simulink model "AC_Capacity_Estimation_Model_AT"  (R2024a)
settings: Solver=FixedStepAuto  StartTime=503  StopTime=2309  FixedStep=0.1  RelTol=1e-3
values from neighbouring files (symbols this model uses):
  airDensity = 1.165    [AC_Capacity_Estimation_Model_Parameters.m]
  airDragCoeff = 0.558    [AC_Capacity_Estimation_Model_Parameters.m]
  frontalArea = 0.958    [AC_Capacity_Estimation_Model_Parameters.m]
  g = 9.8    [AC_Capacity_Estimation_Model_Parameters.m]
  rollingResistCoeff = 0.030    (= 0.03)    [AC_Capacity_Estimation_Model_Parameters.m]
  vehicleMass = 284    [AC_Capacity_Estimation_Model_Parameters.m]
settings Model: Creator=salaz  LastModifiedBy=aimee
settings RTWCC: GPUComputeCapability=3.5

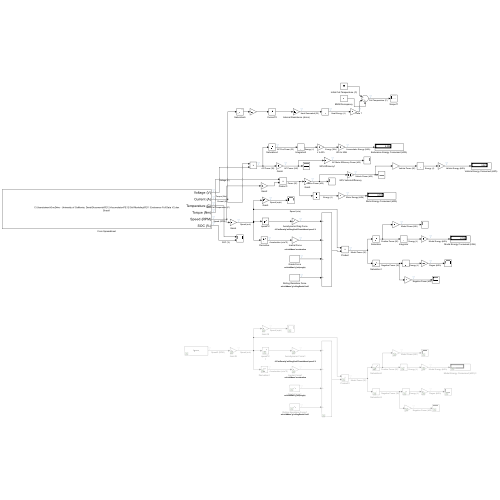
[thumbnail: Simulink's stored preview of the top-level diagram]
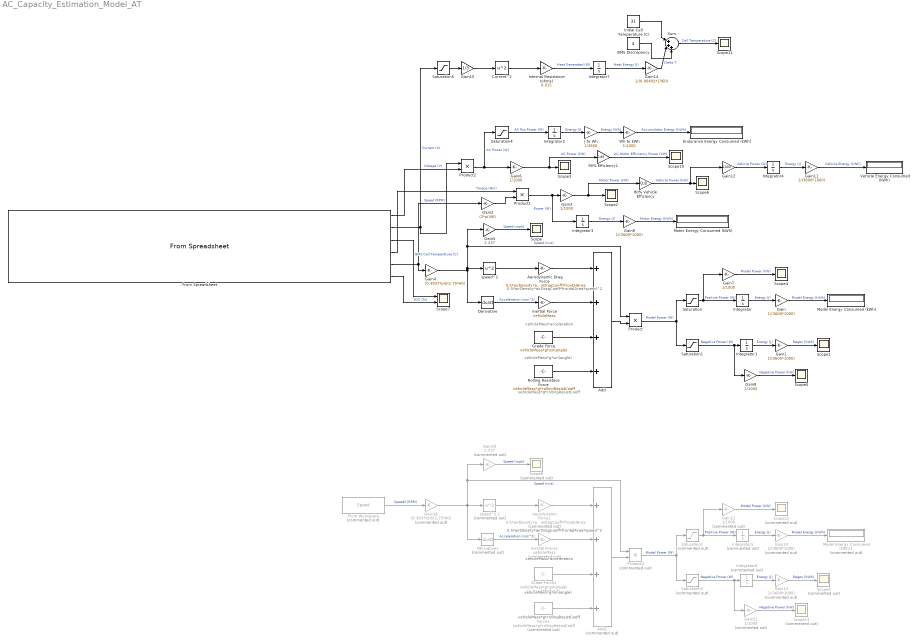
== system AC_Capacity_Estimation_Model_AT ==
  note: 0.5*airDensity*airDragCoeff*frontalArea*speed^2
  note: vehicleMass*acceleration
  note: vehicleMass*g*sin(angle)
  note: vehicleMass*g*rollingResistCoeff
  note: 0.5*airDensity*airDragCoeff*frontalArea*speed^2
  note: vehicleMass*acceleration
  note: vehicleMass*g*sin(angle)
  note: vehicleMass*g*rollingResistCoeff
  80% Vehicle Efficiency : Gain  Gain=0.8
  90% Efficiency1 : Gain  Gain=0.85
  Add : Sum  Inputs=++++
  Add1 : Sum  Commented=on  Inputs=++++
  Aerodynamic Drag Force : Gain  Gain=0.5*airDensity*airDragCoeff*frontalArea
  Aerodynamic Force1 : Gain  Commented=on  Gain=0.5*airDensity*airDragCoeff*frontalArea
  BMS Discrepancy : Constant  Value=4
  "Current^2 " : Math  Operator=square
  Derivative : Derivative
  Derivative1 : Derivative  Commented=on
  "Endurance Energy Consumed (kWh) " : Display
  From Workspace : FromWorkspace  Commented=on  VariableName=Speed
  From Spreadsheet : FromSpreadsheet  FileName=C:\Users\aimee\OneDrive - University of California, Davis\Documents\FE12-Accumulator\FE12\Cell Modeling\FE11 Endurance Full Data V2.xlsx
  Gain{,1,9,11} (4 alike) : Gain  Gain=1/(3600*1000)
  Gain10 : Gain  Commented=on  Gain=1/(3600*1000)
  Gain12 : Gain  Gain=1000
  Gain13 : Gain  Commented=on  Gain=1/(3600*1000)
  Gain14 : Gain  Gain=1/(0.06492*1360)
  Gain15 : Gain  Gain=1/3
  Gain18 : Gain  Commented=on  Gain=(0.3937*pi)/(2.75*60)
  Gain19 : Gain  Commented=on  Gain=2.237
  Gain2 : Gain  Gain=(2*pi)/60
  Gain21 : Gain  Commented=on  Gain=1/1000
  Gain22 : Gain  Commented=on  Gain=1/1000
  Gain{3,6..8} (4 alike) : Gain  Gain=1/1000
  Gain4 : Gain  Gain=(0.3937*pi)/(2.75*60)
  Gain5 : Gain  Gain=2.237
  Grade Force : Constant  Value=vehicleMass*g*sin(angle)
  Grade Force1 : Constant  Commented=on  Value=vehicleMass*g*sin(angle)
  Inertial Force : Gain  Gain=vehicleMass
  Inertial Force1 : Gain  Commented=on  Gain=vehicleMass
  Initial Cell Temperature (C) : Constant  Value=31
  Integrator{,1..4,7} (6 alike) : Integrator
  Integrator5 : Integrator  Commented=on
  Integrator6 : Integrator  Commented=on
  Internal Resistance (ohms) : Gain  Gain=0.015
  J to Wh : Gain  Gain=1/3600
  Model Energy Consumed (kWh) : Display
  Model Energy Consumed (kWh)1 : Display  Commented=on
  Motor Energy Consumed (kWh) : Display
  Product : Product
  Product1 : Product
  Product2 : Product
  Product3 : Product  Commented=on
  Rolling Resistace Force : Constant  Value=vehicleMass*g*rollingResistCoeff
  Rolling Resistace Force1 : Constant  Commented=on  Value=vehicleMass*g*rollingResistCoeff
  Saturation : Saturate  UpperLimit=10^10  LowerLimit=0
  Saturation1 : Saturate  UpperLimit=0  LowerLimit=-10^10
  Saturation2 : Saturate  Commented=on  UpperLimit=10^10  LowerLimit=0
  Saturation3 : Saturate  Commented=on  UpperLimit=0  LowerLimit=-10^10
  Saturation4 : Saturate  UpperLimit=10^10  LowerLimit=0
  Saturation5 : Saturate  UpperLimit=10^10  LowerLimit=0
  Scope{,1..6,10..11} (9 alike) : Scope
  Scope{8..9,12..13} (4 alike) : Scope  Commented=on
  Scope7 : Scope  NumInputPorts=2
  Sum : Sum  Inputs=|+++
  Vehicle Energy Consumed (kWh) : Display
  Wh to kWh : Gain  Gain=1/1000
  "speed^2 " : Math  Operator=square
  speed^2 1 : Math  Commented=on  Operator=square
  wires:
  Gain5/1 -> Scope/1  "Speed (mph)"
  Gain4/1 -> Product/1, Gain5/1, "speed^2 "/1, Derivative/1  "Speed (m/s)"
  Derivative/1 -> Inertial Force/1  "Acceleration (m/s^2)"
  From Spreadsheet/5 -> Gain4/1, Gain2/1  "Speed (RPM)"
  "speed^2 "/1 -> Aerodynamic Drag Force/1
  Aerodynamic Drag Force/1 -> Add/1
  Inertial Force/1 -> Add/2
  Grade Force/1 -> Add/3
  Rolling Resistace Force/1 -> Add/4
  Add/1 -> Product/2
  Product/1 -> Saturation1/1, Saturation/1  "Model Power (W)"
  Saturation/1 -> Gain7/1, Integrator/1  "Positive Power (W)"
  Saturation1/1 -> Integrator1/1, Gain8/1  "Negative Power (W)"
  Integrator/1 -> Gain/1  "Energy (J)"
  Gain/1 -> Model Energy Consumed (kWh)/1  "Model Energy (kWh)"
  Integrator1/1 -> Gain1/1  "Energy (J)"
  Gain1/1 -> Scope1/1  "Regen (kWh)"
  Gain2/1 -> Product1/2
  Gain3/1 -> 80% Vehicle Efficiency/1, Scope2/1  "Motor Power (kW)"
  Product1/1 -> Integrator3/1, Gain3/1  "Power (W)"
  From Spreadsheet/4 -> Product1/1  "Torque (Nm)"
  From Spreadsheet/2 -> Product2/1, Saturation5/1  "Current (A)"
  Gain6/1 -> 90% Efficiency1/1, Scope3/1  "AC Power (kW)"
  Integrator2/1 -> J to Wh/1  "Energy (J)"
  Product2/1 -> Gain6/1, Saturation4/1  "AC Power (W)"
  Wh to kWh/1 -> "Endurance Energy Consumed (kWh) "/1  "Accumulator Energy (kWh)"
  J to Wh/1 -> Wh to kWh/1  "Energy (Wh)"
  From Spreadsheet/1 -> Product2/2  "Voltage (V)"
  Gain7/1 -> Scope4/1  "Model Power (kW)"
  Gain8/1 -> Scope5/1  "Negative Power (kW)"
  Integrator3/1 -> Gain9/1  "Energy (J)"
  Gain9/1 -> Motor Energy Consumed (kWh)/1  "Motor Energy (kWh)"
  80% Vehicle Efficiency/1 -> Gain12/1, Scope6/1  "Vehicle Power (kW)"
  Integrator4/1 -> Gain11/1  "Energy (J)"
  Gain11/1 -> Vehicle Energy Consumed (kWh)/1  "Vehicle Energy (kWh)"
  Gain12/1 -> Integrator4/1  "Vehicle Power (W)"
  From Spreadsheet/6 -> Scope7/2  "SOC (%)"
  Gain22/1 -> Scope13/1  "Negative Power (kW)"
  Gain21/1 -> Scope12/1  "Model Power (kW)"
  Gain13/1 -> Scope9/1  "Regen (kWh)"
  Integrator6/1 -> Gain13/1  "Energy (J)"
  Gain10/1 -> Model Energy Consumed (kWh)1/1  "Model Energy (kWh)"
  Integrator5/1 -> Gain10/1  "Energy (J)"
  Saturation3/1 -> Gain22/1, Integrator6/1  "Negative Power (W)"
  Saturation2/1 -> Integrator5/1, Gain21/1  "Positive Power (W)"
  Product3/1 -> Saturation2/1, Saturation3/1  "Model Power (W)"
  Add1/1 -> Product3/2
  Rolling Resistace Force1/1 -> Add1/4
  Grade Force1/1 -> Add1/3
  Inertial Force1/1 -> Add1/2
  Aerodynamic Force1/1 -> Add1/1
  speed^2 1/1 -> Aerodynamic Force1/1
  From Workspace/1 -> Gain18/1  "Speed2 (RPM)"
  Derivative1/1 -> Inertial Force1/1  "Acceleration (m/s^2)"
  Gain18/1 -> Derivative1/1, speed^2 1/1, Gain19/1, Product3/1  "Speed (m/s)"
  Gain19/1 -> Scope8/1  "Speed (mph)"
  Saturation4/1 -> Integrator2/1  "AC Pos Power (W)"
  90% Efficiency1/1 -> Scope10/1  "AC-Motor Efficiency Power (kW)"
  "Current^2 "/1 -> Internal Resistance (ohms)/1
  Internal Resistance (ohms)/1 -> Integrator7/1  "Heat Generated (W)"
  Integrator7/1 -> Gain14/1  "Heat Energy (J)"
  Gain14/1 -> Sum/2  "Delta T"
  Initial Cell Temperature (C)/1 -> Sum/1
  Sum/1 -> Scope11/1  "Cell Temperature (C)"
  Gain15/1 -> "Current^2 "/1
  Saturation5/1 -> Gain15/1
  From Spreadsheet/3 -> Scope7/1  "BMS Cell Temperature (C)"
  BMS Discrepancy/1 -> Sum/3
